simulink model "model"  (R2024b)
settings: Solver=VariableStepAuto  StartTime=0.0  StopTime=10.0  RelTol=1e-3
values from neighbouring files (symbols this model uses):
  K = acker(A,B,poles_cont)    [startup.m]
  Nu = feedforward_gains(3)    [startup.m]
  Nx = feedforward_gains(1:2)    [startup.m]
  obssysd = c2d(obssys, ts, 'zoh')    [startup.m]
  ts = 0.0001    [startup.m]
undefined symbols (not defined in the file or in its folder): A, B, C, D
settings Model: Creator=Nihal  LastModifiedBy=Nihal

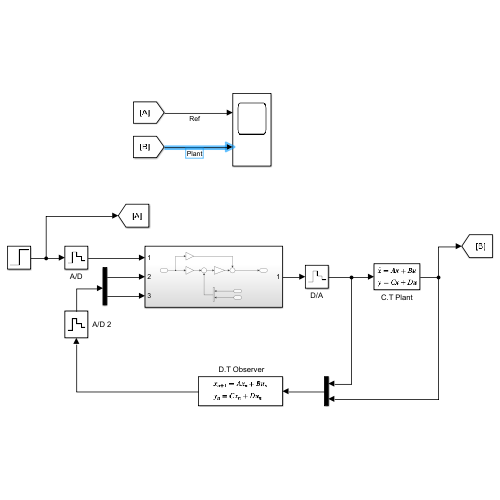
[thumbnail: Simulink's stored preview of the top-level diagram]
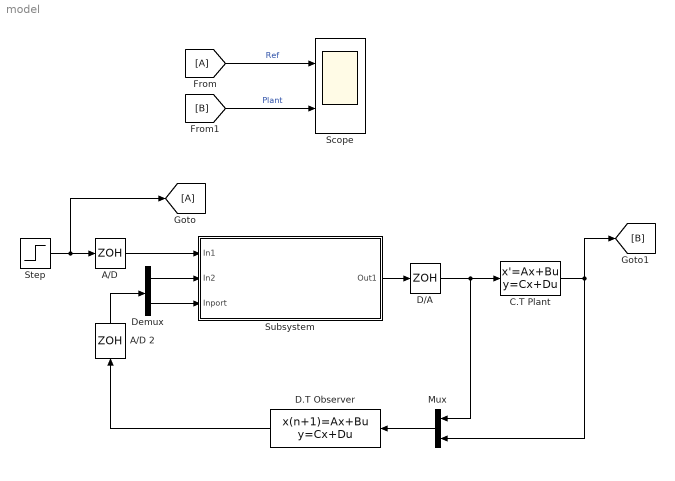
== system model ==
  " D.T Observer" : DiscreteStateSpace  A=obssysd.A  B=obssysd.C  C=obssysd.B  D=obssysd.D  SampleTime=ts
  A/D : ZeroOrderHold  SampleTime=ts
  A/D 2 : ZeroOrderHold  SampleTime=ts
  C.T Plant : StateSpace  A=A  B=B  C=C  D=D  InitialCondition=0
  D/A : ZeroOrderHold  SampleTime=ts
  Demux : Demux  Outputs=2
  From : From
  Goto : Goto
  Mux : Mux  Inputs=2
  Scope : Scope  NumInputPorts=2
  Step : Step  After=40  SampleTime=0
  Subsystem : Subsystem
  wires:
  Demux/1 -> Subsystem/2(In2)
  Demux/2 -> Subsystem/3(Inport)
  " D.T Observer"/1 -> A/D 2/1
  Step/1 -> Goto/1, A/D/1
  A/D/1 -> Subsystem/1(In1)
  A/D 2/1 -> Demux/1
  Subsystem/1(Out1) -> D/A/1
  D/A/1 -> Mux/1, C.T Plant/1
  Mux/1 -> " D.T Observer"/1
  C.T Plant/1 -> Mux/2, [B]
  From/1 -> Scope/1  "Ref"
  [B] -> Scope/2  "Plant"

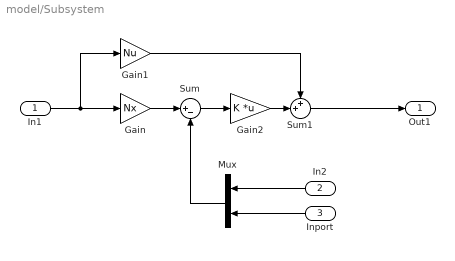
== system model/Subsystem ==
  In1 : Inport
  In2 : Inport  Port=2
  Inport : Inport  Port=3
  Gain : Gain  Gain=Nx
  Gain1 : Gain  Gain=Nu
  Gain2 : Gain  Gain=K  Multiplication=Matrix(K*u)
  Mux : Mux  Inputs=2
  Sum : Sum  Inputs=|+-
  Sum1 : Sum  Inputs=++|
  Out1 : Outport
  wires:
  In1/1 -> Gain1/1, Gain/1
  Gain/1 -> Sum/1
  Mux/1 -> Sum/2
  Sum/1 -> Gain2/1
  Gain2/1 -> Sum1/2
  Gain1/1 -> Sum1/1
  Sum1/1 -> Out1/1
  In2/1 -> Mux/1
  Inport/1 -> Mux/2
